simulink model "Project03_Final"  (R2020b)
settings: Solver=VariableStepAuto  StartTime=0.0  StopTime=5  FixedStep=0.05  RelTol=1e-3
values from neighbouring files (symbols this model uses):
  P_goal = [0.15; 0.02; 0.05]    [run_sim.m]
  P_intermediate = [0.1; 0.01; 0.04]    [run_sim.m]
  P_start = [0; 0; 0]    [run_sim.m]
  simulation_time = 6    [run_sim.m]
libraries: pid_lib x3
settings Model: Creator=berke  LastModifiedBy=berke

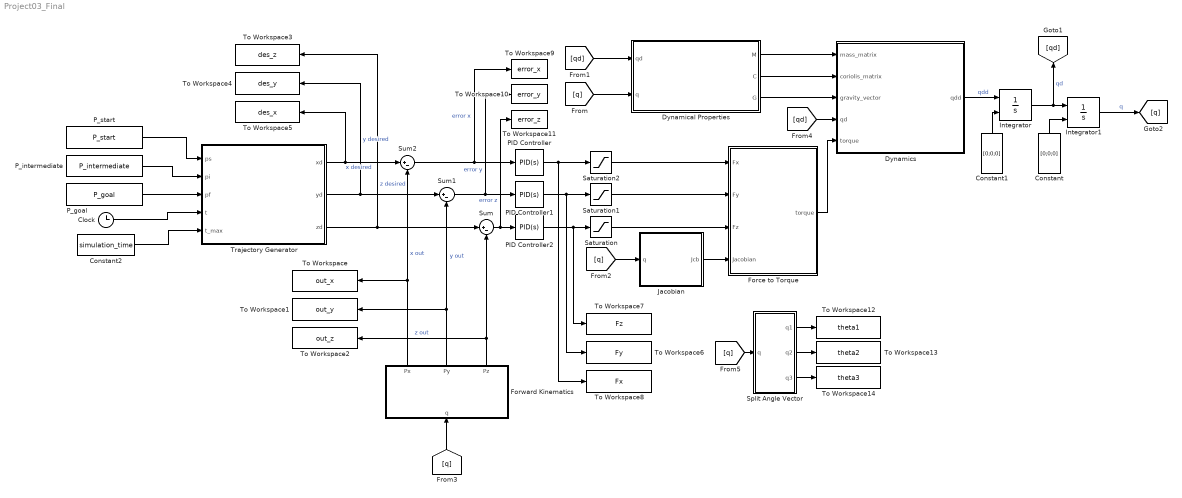
== system Project03_Final ==
  Clock : Clock
  Constant : Constant  Value=[0;0;0]  VectorParams1D=off
  Constant1 : Constant  Value=[0;0;0]  VectorParams1D=off
  Constant2 : Constant  Value=simulation_time
  Dynamical Properties : MATLAB Function  TreatAsAtomicUnit=on
  Dynamics : MATLAB Function  TreatAsAtomicUnit=on
  Force to Torque : MATLAB Function  TreatAsAtomicUnit=on
  Forward Kinematics : MATLAB Function  TreatAsAtomicUnit=on
  Integrator : Integrator  InitialConditionSource=external  InitialCondition=[0;0;0]
  Integrator1 : Integrator  InitialConditionSource=external
  Jacobian : MATLAB Function  TreatAsAtomicUnit=on
  PID Controller : pid_lib/PID Controller  Controller=PID  Form=Parallel  TimeDomain=Continuous-time  UseExternalTs=off  SampleTime=-1  IntegratorMethod=Forward Euler  FilterMethod=Forward Euler  ControllerParametersSource=internal  P=150  I=40  D=40  UseFilter=on  N=100  TunerSelectOption=Transfer Function Based (PID Tuner App)  InitialConditionSource=internal  InitialConditionForIntegrator=0  InitialConditionForFilter=0  DifferentiatorICPrevScaledInput=0  ExternalReset=none  TrackingMode=off  Kt=1  LimitOutput=off  SatLimitsSource=internal  UpperSaturationLimit=inf  LowerSaturationLimit=-inf  LinearizeAsGain=on  AntiWindupMode=none  Kb=1  POutMin=[]  POutMax=[]  IOutMin=[]  IOutMax=[]  DOutMin=[]  DOutMax=[]  NOutMin=[]  NOutMax=[]  SumOutMin=[]  SumOutMax=[]  SaturationOutMin=[]  SaturationOutMax=[]  PParamMin=[]  PParamMax=[]  IParamMin=[]  IParamMax=[]  DParamMin=[]  DParamMax=[]  NParamMin=[]  NParamMax=[]  KbParamMin=[]  KbParamMax=[]  KtParamMin=[]  KtParamMax=[]  KbOutMin=[]  KbOutMax=[]  KtOutMin=[]  KtOutMax=[]  IntegratorOutMin=[]  IntegratorOutMax=[]  FilterOutMin=[]  FilterOutMax=[]  SumI1OutMin=[]  SumI1OutMax=[]  SumI2OutMin=[]  SumI2OutMax=[]  SumI3OutMin=[]  SumI3OutMax=[]  SumI4OutMin=[]  SumI4OutMax=[]  SumDOutMin=[]  SumDOutMax=[]  DifferentiatorOutMin=[]  DifferentiatorOutMax=[]  FilterDiffOutCoefMin=[]  FilterDiffOutCoefMax=[]  ReciprocalOutMin=[]  ReciprocalOutMax=[]  SumDenOutMin=[]  SumDenOutMax=[]  SumNumOutMin=[]  SumNumOutMax=[]  DivideOutMin=[]  DivideOutMax=[]  UdiffTsProdOutMin=[]  UdiffTsProdOutMax=[]  NTsProdOutMin=[]  NTsProdOutMax=[]  UintegralTsProdOutMin=[]  UintegralTsProdOutMax=[]  UngainTsProdOutMin=[]  UngainTsProdOutMax=[]  IntegratorContinuousStateAttributes=''  IntegratorStateMustResolveToSignalObject=off  IntegratorRTWStateStorageClass=Auto  FilterContinuousStateAttributes=''  FilterStateMustResolveToSignalObject=off  FilterRTWStateStorageClass=Auto  ParallelPVariant=InternalParameters  IdealPVariant=Disabled  IVariant=InternalParameters  DVariant=InternalParameters  IntegratorVariant=Continuous  SatVariant=Disabled  AWVariant=Passthrough  PCopyVariant=Disabled  TRVariant=Disabled  FdbkBlocksVariant=Forward  IdealPFdbkVariant=Disabled  SatFdbkVariant=Disabled  DerivativeFilterVariant=ContFilter  NVariant=InternalParameters  NCopyVariant=Disabled  FilterICVariant=InternalICsFilter  IntegratorICVariant=InternalICs  ExternalResetVariant=Disabled  TRSumVariant=Passthrough  SumFdbkVariant=Disabled  SumVariant=Sum_PID  TsampFilterVariant=InternalTs  TsampNgainVariant=Passthrough  TsampIntegralVariant=Passthrough  ExternalSaturationOutDataTypeStr=Inherit: Same as second input
  PID Controller1 : pid_lib/PID Controller  Controller=PID  Form=Parallel  TimeDomain=Continuous-time  UseExternalTs=off  SampleTime=-1  IntegratorMethod=Forward Euler  FilterMethod=Forward Euler  ControllerParametersSource=internal  P=150  I=40  D=40  UseFilter=on  N=100  TunerSelectOption=Transfer Function Based (PID Tuner App)  InitialConditionSource=internal  InitialConditionForIntegrator=0  InitialConditionForFilter=0  DifferentiatorICPrevScaledInput=0  ExternalReset=none  TrackingMode=off  Kt=1  LimitOutput=off  SatLimitsSource=internal  UpperSaturationLimit=inf  LowerSaturationLimit=-inf  LinearizeAsGain=on  AntiWindupMode=none  Kb=1  POutMin=[]  POutMax=[]  IOutMin=[]  IOutMax=[]  DOutMin=[]  DOutMax=[]  NOutMin=[]  NOutMax=[]  SumOutMin=[]  SumOutMax=[]  SaturationOutMin=[]  SaturationOutMax=[]  PParamMin=[]  PParamMax=[]  IParamMin=[]  IParamMax=[]  DParamMin=[]  DParamMax=[]  NParamMin=[]  NParamMax=[]  KbParamMin=[]  KbParamMax=[]  KtParamMin=[]  KtParamMax=[]  KbOutMin=[]  KbOutMax=[]  KtOutMin=[]  KtOutMax=[]  IntegratorOutMin=[]  IntegratorOutMax=[]  FilterOutMin=[]  FilterOutMax=[]  SumI1OutMin=[]  SumI1OutMax=[]  SumI2OutMin=[]  SumI2OutMax=[]  SumI3OutMin=[]  SumI3OutMax=[]  SumI4OutMin=[]  SumI4OutMax=[]  SumDOutMin=[]  SumDOutMax=[]  DifferentiatorOutMin=[]  DifferentiatorOutMax=[]  FilterDiffOutCoefMin=[]  FilterDiffOutCoefMax=[]  ReciprocalOutMin=[]  ReciprocalOutMax=[]  SumDenOutMin=[]  SumDenOutMax=[]  SumNumOutMin=[]  SumNumOutMax=[]  DivideOutMin=[]  DivideOutMax=[]  UdiffTsProdOutMin=[]  UdiffTsProdOutMax=[]  NTsProdOutMin=[]  NTsProdOutMax=[]  UintegralTsProdOutMin=[]  UintegralTsProdOutMax=[]  UngainTsProdOutMin=[]  UngainTsProdOutMax=[]  IntegratorContinuousStateAttributes=''  IntegratorStateMustResolveToSignalObject=off  IntegratorRTWStateStorageClass=Auto  FilterContinuousStateAttributes=''  FilterStateMustResolveToSignalObject=off  FilterRTWStateStorageClass=Auto  ParallelPVariant=InternalParameters  IdealPVariant=Disabled  IVariant=InternalParameters  DVariant=InternalParameters  IntegratorVariant=Continuous  SatVariant=Disabled  AWVariant=Passthrough  PCopyVariant=Disabled  TRVariant=Disabled  FdbkBlocksVariant=Forward  IdealPFdbkVariant=Disabled  SatFdbkVariant=Disabled  DerivativeFilterVariant=ContFilter  NVariant=InternalParameters  NCopyVariant=Disabled  FilterICVariant=InternalICsFilter  IntegratorICVariant=InternalICs  ExternalResetVariant=Disabled  TRSumVariant=Passthrough  SumFdbkVariant=Disabled  SumVariant=Sum_PID  TsampFilterVariant=InternalTs  TsampNgainVariant=Passthrough  TsampIntegralVariant=Passthrough  ExternalSaturationOutDataTypeStr=Inherit: Same as second input
  PID Controller2 : pid_lib/PID Controller  Controller=PID  Form=Parallel  TimeDomain=Continuous-time  UseExternalTs=off  SampleTime=-1  IntegratorMethod=Forward Euler  FilterMethod=Forward Euler  ControllerParametersSource=internal  P=150  I=40  D=40  UseFilter=on  N=100  TunerSelectOption=Transfer Function Based (PID Tuner App)  InitialConditionSource=internal  InitialConditionForIntegrator=0  InitialConditionForFilter=0  DifferentiatorICPrevScaledInput=0  ExternalReset=none  TrackingMode=off  Kt=1  LimitOutput=off  SatLimitsSource=internal  UpperSaturationLimit=inf  LowerSaturationLimit=-inf  LinearizeAsGain=on  AntiWindupMode=none  Kb=1  POutMin=[]  POutMax=[]  IOutMin=[]  IOutMax=[]  DOutMin=[]  DOutMax=[]  NOutMin=[]  NOutMax=[]  SumOutMin=[]  SumOutMax=[]  SaturationOutMin=[]  SaturationOutMax=[]  PParamMin=[]  PParamMax=[]  IParamMin=[]  IParamMax=[]  DParamMin=[]  DParamMax=[]  NParamMin=[]  NParamMax=[]  KbParamMin=[]  KbParamMax=[]  KtParamMin=[]  KtParamMax=[]  KbOutMin=[]  KbOutMax=[]  KtOutMin=[]  KtOutMax=[]  IntegratorOutMin=[]  IntegratorOutMax=[]  FilterOutMin=[]  FilterOutMax=[]  SumI1OutMin=[]  SumI1OutMax=[]  SumI2OutMin=[]  SumI2OutMax=[]  SumI3OutMin=[]  SumI3OutMax=[]  SumI4OutMin=[]  SumI4OutMax=[]  SumDOutMin=[]  SumDOutMax=[]  DifferentiatorOutMin=[]  DifferentiatorOutMax=[]  FilterDiffOutCoefMin=[]  FilterDiffOutCoefMax=[]  ReciprocalOutMin=[]  ReciprocalOutMax=[]  SumDenOutMin=[]  SumDenOutMax=[]  SumNumOutMin=[]  SumNumOutMax=[]  DivideOutMin=[]  DivideOutMax=[]  UdiffTsProdOutMin=[]  UdiffTsProdOutMax=[]  NTsProdOutMin=[]  NTsProdOutMax=[]  UintegralTsProdOutMin=[]  UintegralTsProdOutMax=[]  UngainTsProdOutMin=[]  UngainTsProdOutMax=[]  IntegratorContinuousStateAttributes=''  IntegratorStateMustResolveToSignalObject=off  IntegratorRTWStateStorageClass=Auto  FilterContinuousStateAttributes=''  FilterStateMustResolveToSignalObject=off  FilterRTWStateStorageClass=Auto  ParallelPVariant=InternalParameters  IdealPVariant=Disabled  IVariant=InternalParameters  DVariant=InternalParameters  IntegratorVariant=Continuous  SatVariant=Disabled  AWVariant=Passthrough  PCopyVariant=Disabled  TRVariant=Disabled  FdbkBlocksVariant=Forward  IdealPFdbkVariant=Disabled  SatFdbkVariant=Disabled  DerivativeFilterVariant=ContFilter  NVariant=InternalParameters  NCopyVariant=Disabled  FilterICVariant=InternalICsFilter  IntegratorICVariant=InternalICs  ExternalResetVariant=Disabled  TRSumVariant=Passthrough  SumFdbkVariant=Disabled  SumVariant=Sum_PID  TsampFilterVariant=InternalTs  TsampNgainVariant=Passthrough  TsampIntegralVariant=Passthrough  ExternalSaturationOutDataTypeStr=Inherit: Same as second input
  P_goal : Constant  Value=P_goal  VectorParams1D=off
  P_intermediate : Constant  Value=P_intermediate  VectorParams1D=off
  P_start : Constant  Value=P_start  VectorParams1D=off
  Saturation : Saturate
  Saturation1 : Saturate
  Saturation2 : Saturate
  Split Angle Vector : MATLAB Function  TreatAsAtomicUnit=on
  Sum : Sum  Inputs=|+-
  Sum1 : Sum  Inputs=|+-
  Sum2 : Sum  Inputs=|+-
  To Workspace : ToWorkspace  VariableName=out_x  SampleTime=-1
  To Workspace1 : ToWorkspace  VariableName=out_y  SampleTime=-1
  To Workspace10 : ToWorkspace  VariableName=error_y  SampleTime=-1
  To Workspace11 : ToWorkspace  VariableName=error_z  SampleTime=-1
  To Workspace12 : ToWorkspace  VariableName=theta1  SampleTime=-1
  To Workspace13 : ToWorkspace  VariableName=theta2  SampleTime=-1
  To Workspace14 : ToWorkspace  VariableName=theta3  SampleTime=-1
  To Workspace2 : ToWorkspace  VariableName=out_z  SampleTime=-1
  To Workspace3 : ToWorkspace  VariableName=des_z  SampleTime=-1
  To Workspace4 : ToWorkspace  VariableName=des_y  SampleTime=-1
  To Workspace5 : ToWorkspace  VariableName=des_x  SampleTime=-1
  To Workspace6 : ToWorkspace  VariableName=Fy  SampleTime=-1
  To Workspace7 : ToWorkspace  VariableName=Fz  SampleTime=-1
  To Workspace8 : ToWorkspace  VariableName=Fx  SampleTime=-1
  To Workspace9 : ToWorkspace  VariableName=error_x  SampleTime=-1
  Trajectory Generator : MATLAB Function  TreatAsAtomicUnit=on
  wires:
  Clock/1 -> Trajectory Generator/4(t)
  Forward Kinematics/1(Px) -> Sum2/2, To Workspace/1  "x out"
  Forward Kinematics/2(Py) -> To Workspace1/1, Sum1/2  "y out"
  Forward Kinematics/3(Pz) -> Sum/2, To Workspace2/1  "z out"
  Saturation1/1 -> Force to Torque/2(Fy)
  Saturation2/1 -> Force to Torque/1(Fx)
  Saturation/1 -> Force to Torque/3(Fz)
  Jacobian/1(Jcb) -> Force to Torque/4(Jacobian)
  [q] -> Jacobian/1(q)
  [q] -> Forward Kinematics/1(q)
  P_start/1 -> Trajectory Generator/1(ps)
  P_goal/1 -> Trajectory Generator/3(pf)
  P_intermediate/1 -> Trajectory Generator/2(pi)
  Trajectory Generator/1(xd) -> Sum2/1, To Workspace5/1  "x desired"
  Trajectory Generator/2(yd) -> Sum1/1, To Workspace4/1  "y desired"
  Trajectory Generator/3(zd) -> Sum/1, To Workspace3/1  "z desired"
  Sum2/1 -> To Workspace9/1, PID Controller/1  "error x"
  Sum1/1 -> PID Controller1/1, To Workspace10/1  "error y"
  Sum/1 -> To Workspace11/1, PID Controller2/1  "error z"
  PID Controller/1 -> To Workspace8/1, Saturation2/1
  PID Controller1/1 -> To Workspace6/1, Saturation1/1
  PID Controller2/1 -> To Workspace7/1, Saturation/1
  Constant1/1 -> Integrator/2
  Force to Torque/1(torque) -> Dynamics/5(torque)
  [qd] -> Dynamics/4(qd)
  [qd] -> Dynamical Properties/1(qd)
  Dynamical Properties/1(M) -> Dynamics/1(mass_matrix)
  Dynamics/1(qdd) -> Integrator/1  "qdd"
  Dynamical Properties/2(C) -> Dynamics/2(coriolis_matrix)
  Constant/1 -> Integrator1/2
  Dynamical Properties/3(G) -> Dynamics/3(gravity_vector)
  Integrator/1 -> [qd], Integrator1/1  "qd"
  Integrator1/1 -> [q]  "q"
  [q] -> Dynamical Properties/2(q)
  Constant2/1 -> Trajectory Generator/5(t_max)
  Split Angle Vector/1(q1) -> To Workspace12/1
  Split Angle Vector/3(q3) -> To Workspace14/1
  Split Angle Vector/2(q2) -> To Workspace13/1
  [q] -> Split Angle Vector/1(q)

== matlab function Project03_Final/Dynamics ==
  data: mass_matrix input; qdd output; coriolis_matrix input; gravity_vector input; qd input; torque input
function  qdd = rigid_body_dynamics(mass_matrix, coriolis_matrix, gravity_vector, qd,torque)

qdd = inv(mass_matrix) * (torque - coriolis_matrix * qd - gravity_vector);

== matlab function Project03_Final/Dynamical Properties ==
  data: qd input; q input; M output; C output; G output
function [M,C,G] = dynamical_properties(qd,q)

q1 = q(1); q2 = q(2); q3 = q(3); 
q1d = qd(1); q2d = qd(2); q3d = qd(3); 

%% phantom premium 1.5 parameters
ma = 0.0202;%new
mc = 0.0249;%new
mbe = 0.2359;%new
mdf = 0.1906;
l1 = 0.215;%new
l2 = 0.170;
l3 = 0.0325;
l5 = -36.8e-3;
l6 = 52.7e-3;
g = 9.81;

%% moment of inertia params
Iaxx = 0.4864e-4;
Iayy = 0.001843e-4;
Iazz = 0.4864e-4;
Icxx = 0.959e-4;
Icyy = 0.959e-4;
Iczz = 0.0051e-4;
Ibexx = 11.09e-4;
Ibeyy = 10.06e-4;
Ibezz = 0.591e-4;
Idfxx = 7.11e-4;
Idfyy = 0.629e-4;
Idfzz = 6.246e-4;
Ibaseyy = 11.87e-4;

%% mass matrix components
m11 = (0.125*(4*Iayy+4*Iazz+8*Ibaseyy+4*Ibeyy+4*Ibezz+4*Icyy+4*Iczz+4*Idfyy+4*Idfzz+4*l1*l1*ma+l2*l2*ma+l1*l1*mc+4*l3*l3*mc)...
    +0.125*(4*Ibeyy-4*Ibezz+4*Icyy-4*Iczz+l1*l1*(4*ma+mc))*cos(2*q2)...
    +0.125*(4*Iayy-4*Iazz+4*Idfyy-4*Idfzz-l2*l2*ma-4*l3*l3*mc)*cos(2*q3)+l1*(l2*ma+l3*mc)*cos(q2)*sin(q3));
m22 = 0.25*(4*(Ibexx+Icxx+l1*l1*ma)+l1*l1*mc);
m23 = -0.5*l1*(l2*ma+l3*mc)*sin(q2-q3);
m32 = m23;
m33 = 0.25*(4*Iaxx+4*Idfxx+l2*l2*ma+4*l3*l3*mc);

M = [m11 0 0;
    0 m22 m23;
    0 m32 m33];


%% coriolis matrix components
c11 = 0.125*(-2*sin(q2)*((4*Ibeyy-4*Ibezz+4*Icyy-4*Iczz+4*l1*l1*ma+l1*l1*mc)*cos(q2)+2*l1*(l2*ma+l3*mc)*sin(q3))*q2d...
    +2*cos(q3)*(2*l1*(l2*ma+l3*mc)*cos(q2)+(-4*Iayy+4*Iazz-4*Idfyy+4*Idfzz+l2*l2*ma+4*l3*l3*mc)*sin(q3))*q3d);
c12 = -0.125*((4*Ibeyy-4*Ibezz+4*Icyy-4*Iczz+l1*l1*(4*ma+mc))*sin(2*q2)+4*l1*(l2*ma+l3*mc)*sin(q2)*sin(q3))*q1d;
c13 = -0.125*(-4*l1*(l2*ma+l3*mc)*cos(q2)*cos(q3)-(-4*Iayy+4*Iazz-4*Idfyy+4*Idfzz+l2*l2*ma+4*l3*l3*mc)*sin(2*q3))*q1d;
c21 = -c12;
c22 = 0;
c23 = 0.5*l1*(l2*ma+l3*mc)*cos(q2-q3)*q3d;
c31 = -c13;
c32 = 0.5*l1*(l2*ma+l3*mc)*cos(q2-q3)*q2d;
c33 = 0;

C = [c11 c12 c13;
    c21 c22 c23;
    c31 c32 c33];

%% gravity vector components
tg1 = 0;
tg2 = g*(l1*(ma+0.5*mc)+l5*mbe)*cos(q2);
tg3 = g*(0.5*l2*ma+l3*mc-l6*mdf)*sin(q3);


G = [0;
    tg2;
    tg3];

== matlab function Project03_Final/Trajectory Generator ==
  data: ps input; pi input; pf input; xd output; yd output; zd output; t input; t_max input
function [xd, yd, zd] = get_path(ps, pi, pf, t, t_max)
% INPUTS
% ps: start point 
% pi: intermediate point     
% pf: final point 
% t : simulation time
    
% OUTPUTS
% xd: x-coordinate of the desired point
% yd: y-coordinate of the desired point
% zd: z-coordinate of the desired point

% t0 is assummed to be the 0th second
 
max_simulation_time = t_max; % Duration of the simulation has to be equal to this number.

via_points_on_path = [ps pi pf]; % Concetenate the input points
number_of_points_on_path = 1001; % Number of points in the trajectory

points_on_path = trapveltraj(via_points_on_path, number_of_points_on_path); % Use the built-in function to generate a linear trajectory

% Map the range [0 max_simulation_time] to [1 number_of_points_on_path].
% Purpose of this mapping is to achieve desired coordinate values with
% equally spaced time increments.
index_of_point = round(t * (number_of_points_on_path - 1) / (max_simulation_time) + 1);                   

% Desired x,y,z coordinates of the end-effector
xd = points_on_path(1,index_of_point); 
yd = points_on_path(2,index_of_point);
zd = points_on_path(3,index_of_point);
end

== matlab function Project03_Final/Forward Kinematics ==
  data: q input; Px output; Py output; Pz output
function [Px,Py,Pz] = forward_kinematics(q)
p = [0,0,0,1];
l1 = 0.215;%new
l2 = 0.170;
T = @(t1, t2, t3)(...
    [cos(t1) -sin(t1)*sin(t3) cos(t3)*sin(t1) sin(t1)*(l1*cos(t2)+l2*cos(t3));...
    0 cos(t3) sin(t3) l2-l2*cos(t3)+l1*sin(t2);...
    -sin(t1) -cos(t1)*sin(t3) cos(t1)*cos(t3) -l1+cos(t1)*(l1*cos(t2)+l2*sin(t3));...
    0 0 0 1]);

t1 = q(1); t2 = q(2); t3 = q(3);
y = T(t1, t2, t3) * p';

Px = y(1);
Py = y(2);
Pz = y(3);
end

== matlab function Project03_Final/Jacobian ==
  data: q input; Jcb output
function Jcb = get_jac(q)
%return the basic Jacobian matrix for the given joint configuration

l1 = 0.215;%new
l2 = 0.170;

Jcb = [...
    l1*cos(q(1))*cos(q(2))+l2*cos(q(1))*sin(q(3)),l1*sin(q(2))*sin(q(1)),l2*cos(q(3))*sin(q(1));
    0,l1*cos(q(2)),l2*sin(q(3));
    -l1*sin(q(1))*cos(q(2))-l2*sin(q(1))*sin(q(3)),-l1*sin(q(2))*cos(q(1)),l2*cos(q(3))*cos(q(1))];

end

== matlab function Project03_Final/Split Angle Vector ==
  data: q input; q1 output; q2 output; q3 output
function [q1,q2,q3] = split_matrix(q)

q1 = q(1);
q2 = q(2);
q3 = q(3);

== matlab function Project03_Final/Force to Torque ==
  data: Fx input; Fy input; Fz input; Jacobian input; torque output
function torque = multiplication(Fx,Fy,Fz,Jacobian)
Force = [Fx; Fy; Fz];

torque = transpose(Jacobian) * Force;
